simulink library "tetherDragForceNGreater2_ul"  (R2018b)
settings: Solver=VariableStepAuto  StartTime=0.0  StopTime=10.0  RelTol=1e-3
values from neighbouring files (symbols this model uses):
  N = 5    [tetherDragForce_ts.m]
settings Model: Creator=asiddiq2  LastModifiedBy=asiddiq2

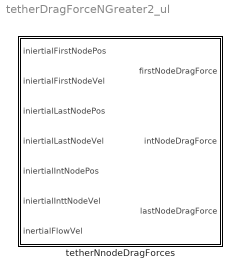
== system tetherDragForceNGreater2_ul ==
  tetherNnodeDragForces : Subsystem  mask{rhoFluid=1, numNode=4, diaTether=1, CdTether=0.5}
      mask prompts: rhoFluid "Fluid density"; numNode "Number of Nodes"; diaTether "Tether diameter"; CdTether "Drag coefficient"
      mask DialogControl Container3 Prompt: Environment
      mask DialogControl ParameterGroupVar Prompt: Tether

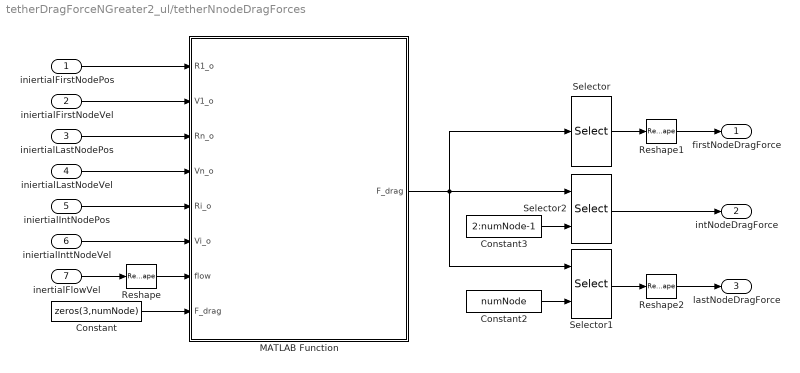
== system tetherDragForceNGreater2_ul/tetherNnodeDragForces ==
  iniertialFirstNodePos : Inport
  iniertialFirstNodeVel : Inport  Port=2
  iniertialLastNodePos : Inport  Port=3
  iniertialLastNodeVel : Inport  Port=4
  iniertialIntNodePos : Inport  Port=5
  iniertialInttNodeVel : Inport  Port=6
  inertialFlowVel : Inport  Port=7
  Constant : Constant  Value=zeros(3,numNode)  VectorParams1D=off
  Constant2 : Constant  Value=numNode  VectorParams1D=off
  Constant3 : Constant  Value=2:numNode-1  VectorParams1D=off
  MATLAB Function : MATLAB Function  TreatAsAtomicUnit=on
  Reshape : Reshape  OutputDimensionality=Column vector (2-D)
  Reshape1 : Reshape  OutputDimensionality=Column vector (2-D)
  Reshape2 : Reshape  OutputDimensionality=Column vector (2-D)
  Selector : Selector  NumberOfDimensions=2  InputPortWidth=3  IndexOptions=Select all,Index vector (dialog)  Indices=[1 3],1  OutputSizes=1,1
  Selector1 : Selector  NumberOfDimensions=2  InputPortWidth=3  IndexOptions=Select all,Index vector (port)  Indices=[1 3],N  OutputSizes=1,1
  Selector2 : Selector  NumberOfDimensions=2  InputPortWidth=3  IndexOptions=Select all,Index vector (port)  Indices=[1 3],[2:N-1]  OutputSizes=1,1
  firstNodeDragForce : Outport
  intNodeDragForce : Outport  Port=2
  lastNodeDragForce : Outport  Port=3
  wires:
  inertialFlowVel/1 -> Reshape/1
  Constant/1 -> MATLAB Function/8("F_drag ")
  Reshape/1 -> MATLAB Function/7(flow)
  iniertialInttNodeVel/1 -> MATLAB Function/6(Vi_o)
  iniertialIntNodePos/1 -> MATLAB Function/5(Ri_o)
  iniertialLastNodeVel/1 -> MATLAB Function/4(Vn_o)
  iniertialLastNodePos/1 -> MATLAB Function/3(Rn_o)
  iniertialFirstNodeVel/1 -> MATLAB Function/2(V1_o)
  iniertialFirstNodePos/1 -> MATLAB Function/1(R1_o)
  Constant3/1 -> Selector2/2
  Constant2/1 -> Selector1/2
  MATLAB Function/1(F_drag) -> Selector2/1, Selector/1, Selector1/1
  Selector2/1 -> intNodeDragForce/1
  Selector1/1 -> Reshape2/1
  Selector/1 -> Reshape1/1
  Reshape1/1 -> firstNodeDragForce/1
  Reshape2/1 -> lastNodeDragForce/1

== matlab function tetherDragForceNGreater2_ul/tetherNnodeDragForces/MATLAB Function ==
  data: R1_o input; V1_o input; Rn_o input; Vn_o input; Ri_o input; F_drag output; Vi_o input; flow input; F_drag input; CdTether parameter; rhoFluid parameter; numNode parameter; diaTether parameter
function F_drag = fcn(R1_o,V1_o,Rn_o,Vn_o,Ri_o,Vi_o,flow,F_drag,...
    CdTether, rhoFluid, numNode,  diaTether)

Ri_o = [R1_o Ri_o Rn_o];
Vi_o = [V1_o Vi_o Vn_o];

Ve = zeros(3,numNode-1);
Vrel = zeros(3,numNode-1);
drag_direction = zeros(3,numNode-1);
drag = zeros(3,numNode-1);

qe = zeros(numNode-1,1);
di = zeros(numNode-1,1);
th = zeros(numNode-1,1);
S = zeros(numNode-1,1);

% elemental velocity
for i = 1:numNode-1
    
    % relative velocity
    Ve(:,i) = (Vi_o(:,i) + Vi_o(:,i+1))/2;
    Vrel(:,i) = flow - Ve(:,i);
    Vrel(3,i) = 0;
    % drag direction
    if norm(Vrel(:,i)) > 1e-3
        drag_direction(:,i) = Vrel(:,i)/norm(Vrel(:,i));
    else
        drag_direction(:,i) = zeros(3,1);
    end
    
    % dynamic pressure
    qe(i) = 0.5*rhoFluid*norm(Vrel(:,i))^2;
    
    % projected area
    di(i) = norm(Ri_o(:,i+1)-Ri_o(:,i));
    th(i) = atan( (Ri_o(3,i+1)-Ri_o(3,i))/norm(Ri_o(1:2,i+1)-Ri_o(1:2,i)) );
    S(i) = di(i)*diaTether*sin(th(i));
    
    drag(:,i) = 0.5*rhoFluid*CdTether*Vrel(:,i)*norm(Vrel(:,i))*S(i);
end

% drag force acting on each node'
for i = 1:numNode
    if i == 1
        F_drag(:,i) = drag(:,i)/2;
    elseif i> 1 && i < numNode
        F_drag(:,i) = (drag(:,i-1) + drag(:,i))/2;
    elseif i == numNode
        F_drag(:,i) = drag(:,i-1)/2;
    end
end

end
